simulink model "Model3"  (R2020a)
settings: Solver=VariableStepAuto  StartTime=0.0  StopTime=80  RelTol=1e-3
undefined symbols (not defined in the file): a, a0, a1, a10, a11, a12, a13, a14, a15, a16, a17, a2, a3, a4, a5, a6, a7, a8, a9, alpha, Area, b, b1, b11, b12, b2, bankingAngle, C_fuel, camber, curveCenters, Cx, Cz, distanceThreshold, g, init_vel, init_y_pos, IT, K_wear, l_f, l_r, m_fuel, mT, overlapThreshold, rho_0, rho_1, TyreContactArea, w1, w2
libraries: simulink x7
(part 1 of 2)
settings Model: PacingRate=2  Creator=carmelo  LastModifiedBy=cvalo

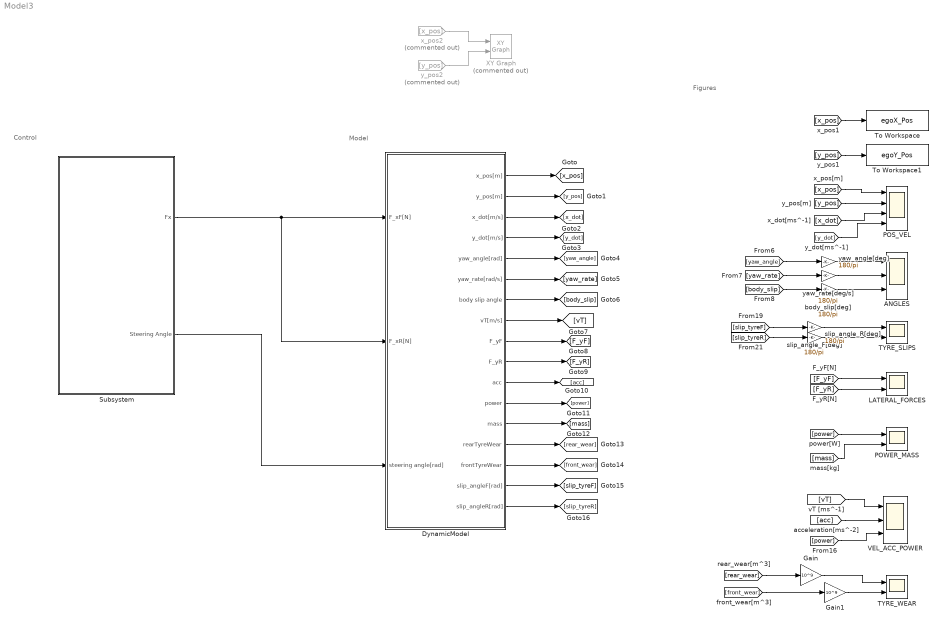
== system Model3 ==
  note: Control
  note: Model
  note: Figures
  ANGLES : Scope  NumInputPorts=3
  DynamicModel : Subsystem
  Gain : Gain  Gain=10^9
  Gain1 : Gain  Gain=10^9
  LATERAL_FORCES : Scope  NumInputPorts=2
  POS_VEL : Scope  NumInputPorts=4
  POWER_MASS : Scope  NumInputPorts=2
  Subsystem : Subsystem
  TYRE_SLIPS : Scope  NumInputPorts=2
  TYRE_WEAR : Scope  NumInputPorts=2
  To Workspace : ToWorkspace  VariableName=egoX_Pos  SampleTime=-1
      settings: Decimation=3
  To Workspace1 : ToWorkspace  VariableName=egoY_Pos  SampleTime=-1
      settings: Decimation=3
  VEL_ACC_POWER : Scope  NumInputPorts=3
  XY Graph : simulink/Sinks/XY Graph  Commented=on  xmin=-1000  xmax=1000  ymin=-1000  ymax=1000  st=-1
  body_slip[deg] : Gain  Gain=180/pi
  slip_angle_F[deg] : Gain  Gain=180/pi
  slip_angle_R[deg] : Gain  Gain=180/pi
  x_pos2 : From  Commented=on  GotoTag=x_pos
  y_pos2 : From  Commented=on  GotoTag=y_pos
  yaw_angle[deg] : Gain  Gain=180/pi
  yaw_rate[deg/s] : Gain  Gain=180/pi
  wires:
  DynamicModel/3(x_dot[m/s]) -> [x_dot]
  DynamicModel/4(y_dot[m/s]) -> [y_dot]
  DynamicModel/1(x_pos[m]) -> [x_pos]
  DynamicModel/2(y_pos[m]) -> [y_pos]
  Subsystem/1(Fx) -> DynamicModel/1(F_xF[N]), DynamicModel/2(F_xR[N])
  Subsystem/2(Steering Angle) -> DynamicModel/3(steering angle[rad])
  DynamicModel/5(yaw_angle[rad]) -> [yaw_angle]
  DynamicModel/6(yaw_rate[rad/s]) -> [yaw_rate]
  DynamicModel/7(body slip angle) -> [body_slip]
  DynamicModel/8(vT[m/s]) -> [vT]
  DynamicModel/9(F_yF) -> [F_yF]
  DynamicModel/10(F_yR) -> [F_yR]
  DynamicModel/11(acc) -> [acc]
  DynamicModel/12(power) -> [power]
  DynamicModel/13(mass) -> [mass]
  DynamicModel/15(frontTyreWear) -> [front_wear]
  DynamicModel/14(rearTyreWear) -> [rear_wear]
  DynamicModel/16(slip_angleF[rad]) -> [slip_tyreF]
  DynamicModel/17(slip_angleR[rad]) -> [slip_tyreR]
  slip_angle_R[deg]/1 -> TYRE_SLIPS/2
  [x_pos] -> POS_VEL/1
  [front_wear] -> Gain1/1
  [mass] -> POWER_MASS/2
  yaw_rate[deg/s]/1 -> ANGLES/2
  body_slip[deg]/1 -> ANGLES/3
  [yaw_angle] -> yaw_angle[deg]/1
  [y_dot] -> POS_VEL/4
  [y_pos] -> POS_VEL/2
  [yaw_rate] -> yaw_rate[deg/s]/1
  [body_slip] -> body_slip[deg]/1
  [power] -> POWER_MASS/1
  [acc] -> VEL_ACC_POWER/2
  [rear_wear] -> Gain/1
  yaw_angle[deg]/1 -> ANGLES/1
  [x_pos] -> To Workspace/1
  [F_yR] -> LATERAL_FORCES/2
  [slip_tyreR] -> slip_angle_R[deg]/1
  [y_pos] -> To Workspace1/1
  [slip_tyreF] -> slip_angle_F[deg]/1
  [F_yF] -> LATERAL_FORCES/1
  [power] -> VEL_ACC_POWER/3
  [x_dot] -> POS_VEL/3
  slip_angle_F[deg]/1 -> TYRE_SLIPS/1
  [vT] -> VEL_ACC_POWER/1
  Gain/1 -> TYRE_WEAR/1
  Gain1/1 -> TYRE_WEAR/2
  x_pos2/1 -> XY Graph/1
  y_pos2/1 -> XY Graph/2

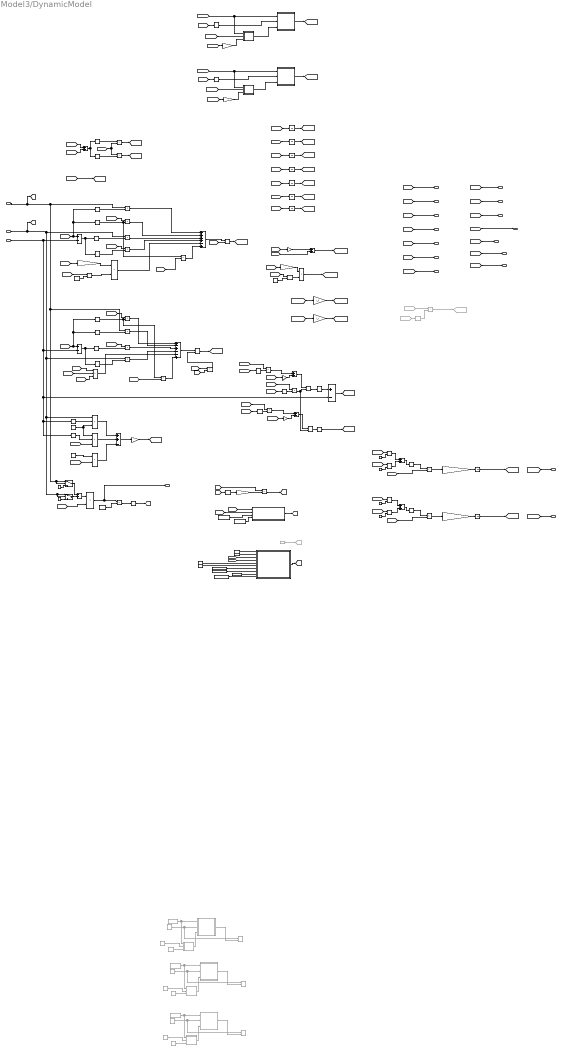
== system Model3/DynamicModel ==
  note: Wind effect
  note: DEBUG
  note: FN
  note: Fx_F
  note: Tyre wears
  note: Outputs
  note: Longitudinal velocity
  note: Outputs
  note: Tires slip angles
  note: Tire lateral forces
  note: x6_dot equation
  note: Continuos integration
  note: x4_dot equation
  note: x3_dot equation
  note: x1_dot and x2_dot equations
  note: x5_dot equation
  note: mdot
  note: vertical force
  note: Fx_R
  F_xF[N] : Inport  Unit=N
  F_xR[N] : Inport  Port=2  Unit=N
  steering angle[rad] : Inport  Port=3  Unit=rad
  Add : Sum
  Add1 : Sum
  Add2 : Sum
  Atan : Trigonometry  Operator=atan
  Atan1 : Trigonometry  Operator=atan
  Calculate Peak : Subsystem
  Calculate Peak1 : Subsystem
  Calculate Peak2 : Subsystem  Commented=on
  Calculate Peak3 : Subsystem  Commented=on
  Calculate Peak4 : Subsystem  Commented=on
  Constant : Constant  Commented=on  Value=0
  Constant1 : Constant  Value=a
  Constant10 : Constant  Value=C_fuel
  Constant{5..6,9,11..12,14} (6 alike) : Constant  Value=2
  Constant13 : Constant  Value=-5.625
  Constant15 : Constant  Commented=on  Value=7500
  Constant16 : Constant  Commented=on  Value=7500
  Constant17 : Constant  Commented=on  Value=1500
  Constant18 : Constant  Commented=on  Value=8000
  Constant19 : Constant  Value=rho_0
  Constant2 : Constant  Value=b
  Constant20 : Constant  Value=rho_1
  Constant21 : Constant  Value=distanceThreshold
  Constant22 : Constant  Value=overlapThreshold
  Constant23 : Constant  Value=curveCenters
  Constant24 : Constant  Value=alpha
  Constant25 : Constant  Commented=on  Value=rho_0
  Constant3 : Constant  Commented=on  Value=4000
  Constant32 : Constant  Value=bankingAngle
  Constant33 : Constant  Value=curveCenters
  Constant34 : Constant  Value=0
  Constant35 : Constant  Value=0
  Constant38 : Constant  Commented=on  Value=7500
  Constant4 : Constant  Commented=on  Value=1500
  Constant7 : Constant  Commented=on  Value=0
  Constant8 : Constant  Value=10
  Cos{,1..6} (7 alike) : Trigonometry  Operator=cos
  Cos7 : Trigonometry  Commented=on  Operator=cos
  Divide{,1..3} (4 alike) : Product  Inputs=*/
  FindBankingData : MATLAB Function  TreatAsAtomicUnit=on
  From37 : From  Commented=on  GotoTag=x4_vT
  From38 : From  Commented=on  GotoTag=x5_slip_angle
  Gain : Gain  Gain=g
  Gain1 : Gain  Gain=K_wear/TyreContactArea
  Gain10 : Gain  Gain=10^9
  Gain11 : Gain  Gain=10^9
  Gain2 : Gain  Gain=1/IT
  Gain21 : Gain  Gain=l_r
  Gain3 : Gain  Gain=K_wear/TyreContactArea
  Gain4 : Gain  Gain=a
  Gain5 : Gain  Gain=b
  Gain6 : Gain  Gain=Area*Cx*0.5
  Gain7 : Gain  Gain=l_f
  Gain8 : Gain  Gain=g
  Gain9 : Gain  Gain=Area*Cz*0.5
  Goto16 : Goto  Commented=on  GotoTag=longitudinal_vel
  Goto22 : Goto  Commented=on  GotoTag=rho
  Integrator{,2,4..5,7..8} (6 alike) : Integrator
  Integrator1 : Integrator  InitialCondition=init_y_pos
  Integrator3 : Integrator  InitialCondition=init_vel
  Integrator6 : Integrator  InitialCondition=mT  LimitOutput=on  UpperSaturationLimit=mT  LowerSaturationLimit=mT - m_fuel
  Minus : Sum  Inputs=+-
  Minus1 : Sum  Inputs=+-
  Minus2 : Sum  Inputs=+-
  PacejkaF : Subsystem
  PacejkaF1 : Subsystem
  PacejkaF2 : Subsystem  Commented=on
  PacejkaF3 : Subsystem  Commented=on
  PacejkaF4 : Subsystem  Commented=on
  Plus : Sum
  Plus1 : Sum  Inputs=++++-+
  Plus2 : Sum  Inputs=+-+--+
  Plus3 : Sum  Inputs=++-
  Plus4 : Sum
  Plus5 : Sum  Inputs=+-
  Plus7 : Sum
  Power{,1..5} (6 alike) : Math  Operator=pow  SaturateOnIntegerOverflow=on
  Product{,1..9,13..16,18..23,25,31,35..36} (24 alike) : Product
  Product10 : Product  Inputs=3
  Product11 : Product  Inputs=3
  Product12 : Product  Inputs=3
  Product17 : Product  Commented=on
  Ramp1 : simulink/Sources/Ramp  Commented=on  slope=0.01  start=0  InitialOutput=0
  Ramp2 : simulink/Sources/Ramp  Commented=on  slope=0.01  start=0  InitialOutput=0
  Ramp6 : simulink/Sources/Ramp  Commented=on  slope=0.01  start=0  InitialOutput=0
  Sin{,1..7,11} (9 alike) : Trigonometry
  Sqrt : Sqrt  SaturateOnIntegerOverflow=on
  Sqrt1 : Sqrt  SaturateOnIntegerOverflow=on
  Switch : Switch
  Switch1 : Switch
  Unary Minus : UnaryMinus
  Unary Minus5 : UnaryMinus
  Unary Minus6 : UnaryMinus
  WindEffect : MATLAB Function  TreatAsAtomicUnit=on
  XY Graph1 : simulink/Sinks/XY Graph  Commented=on  xmin=0  xmax=1  ymin=0  ymax=7000  st=-1
  XY Graph2 : simulink/Sinks/XY Graph  Commented=on  xmin=0  xmax=1  ymin=0  ymax=7000  st=-1
  XY Graph3 : simulink/Sinks/XY Graph  Commented=on  xmin=0  xmax=1  ymin=0  ymax=7000  st=-1
  x_pos[m] : Outport  Unit=m
  y_pos[m] : Outport  Port=2  Unit=m
  x_dot[m/s] : Outport  Port=3  Unit=m/s
  y_dot[m/s] : Outport  Port=4  Unit=m/s
  yaw_angle[rad] : Outport  Port=5  Unit=rad
  yaw_rate[rad/s] : Outport  Port=6  Unit=rad/s
  body slip angle : Outport  Port=7  Unit=rad
  vT[m/s] : Outport  Port=8  Unit=m/s
  F_yF : Outport  Port=9  Unit=N
  F_yR : Outport  Port=10  Unit=N
  acc : Outport  Port=11  Unit=m/s^2
  power : Outport  Port=12  Unit=watt
  mass : Outport  Port=13  Unit=kg
  rearTyreWear : Outport  Port=14  Unit=m^3
  frontTyreWear : Outport  Port=15  Unit=m^3
  slip_angleF[rad] : Outport  Port=16  Unit=rad
  slip_angleR[rad] : Outport  Port=17  Unit=rad
  wires:
  [x5_slip_angle] -> Sin7/1
  [x4_vT] -> Product16/1
  Atan/1 -> Minus2/1
  Product17/1 -> Goto16/1
  [x1_x_pos] -> x_pos[m]/1
  [x6_yaw_rate] -> Gain4/1
  [F_yR] -> Product13/2
  Sin/1 -> Product1/2
  Integrator3/1 -> [x4_vT]
  Cos7/1 -> Product17/2
  Sin2/1 -> Product35/1, Product4/2
  Product4/1 -> Plus1/2
  [x3_dot] -> Integrator2/1
  Divide1/1 -> Atan1/1
  Product2/1 -> Plus1/3
  [F_yF] -> Product6/1
  Product14/1 -> Divide/2, Divide1/2
  [x5_slip_angle] -> Sin2/1, Cos2/1, Minus/1
  Minus2/1 -> [slip_angle_F]
  Cos2/1 -> Product3/2
  [x5_slip_angle] -> Plus/2
  Sin7/1 -> Product16/2
  Integrator5/1 -> [x6_yaw_rate]
  [x4_dot] -> Integrator3/1
  Product/1 -> [x1_dot]
  [x3_yaw_angle] -> yaw_angle[rad]/1
  [x1_dot] -> x_dot[m/s]/1
  Constant2/1 -> Product13/1
  Cos3/1 -> Product6/2
  [x2_dot] -> Integrator1/1
  Minus/1 -> Sin1/1, Cos1/1
  [x6_dot] -> Integrator5/1
  Integrator2/1 -> [x3_yaw_angle]
  Gain4/1 -> Plus4/2
  [x2_y_pos] -> y_pos[m]/1
  Cos1/1 -> Product2/2
  Gain2/1 -> [x6_dot]
  [x4_vT] -> Product10/2
  [x6_yaw_rate] -> [x3_dot]
  [F_yF] -> Product5/1
  [x3_yaw_angle] -> Plus/1
  [x6_yaw_rate] -> yaw_rate[rad/s]/1
  [F_yR] -> Product4/1
  [x4_vT] -> Product15/1
  [x4_vT] -> vT[m/s]/1
  [x5_slip_angle] -> Sin6/1
  Product11/1 -> Plus3/1
  [F_yR] -> Product7/1
  Atan1/1 -> [slip_angle_R]
  Divide/1 -> Atan/1
  [x4_vT] -> Product1/1, Product/2
  Product1/1 -> [x2_dot]
  Cos4/1 -> Product36/1, Product7/2
  Sin5/1 -> Product11/2
  Plus5/1 -> Divide1/1
  [x5_slip_angle] -> Cos6/1
  Sin4/1 -> Product8/2
  [x6_yaw_rate] -> Product10/3
  Cos5/1 -> Product12/2
  Plus3/1 -> Gain2/1
  Cos/1 -> Product/1
  Product13/1 -> Plus3/3
  Cos6/1 -> Product14/2
  Integrator/1 -> [x1_x_pos]
  Plus/1 -> Cos/1, Sin/1
  Product12/1 -> Plus3/2
  Product5/1 -> Plus1/4
  steering angle[rad]/1 -> Minus2/2, Cos5/1, Sin5/1, Minus1/2, Minus/2
  Product15/1 -> Plus4/1
  [x5_dot] -> Integrator4/1
  Product9/1 -> Plus2/4
  Product16/1 -> Plus5/1
  [x4_vT] -> Product14/1
  [mT] -> Product10/1
  From37/1 -> Product17/1
  Sin3/1 -> Product9/2
  Plus2/1 -> Divide2/1
  Product6/1 -> Plus2/3
  [x5_slip_angle] -> Sin4/1, Cos4/1, Minus1/1
  Constant1/1 -> Product11/3, Product12/1
  Divide2/1 -> [x5_dot]
  Integrator1/1 -> [x2_y_pos]
  [F_yF] -> Product12/3
  Minus1/1 -> Sin3/1, Cos3/1
  Product10/1 -> Plus2/5
  Product7/1 -> Plus2/1
  From38/1 -> Cos7/1
  Sin1/1 -> Product5/2
  [x6_yaw_rate] -> Gain5/1
  [x1_dot] -> Integrator/1
  [x2_dot] -> y_dot[m/s]/1
  Product3/1 -> Plus1/1
  Sin6/1 -> Product15/2
  Integrator4/1 -> [x5_slip_angle]
  Product8/1 -> Plus2/2
  Plus4/1 -> Divide/1
  Gain5/1 -> Plus5/2
  Divide3/1 -> [x4_dot]
  Plus1/1 -> Divide3/1
  [F_yF] -> F_yF/1
  [F_yR] -> F_yR/1
  [x5_slip_angle] -> body slip angle/1
  [x4_dot] -> acc/1
  Product18/1 -> Divide2/2
  [mT] -> Product18/1
  [x4_vT] -> Product18/2
  [x4_vT] -> Power/1
  Product19/1 -> Plus1/5
  [rho] -> Gain6/1
  Constant6/1 -> Power/2
  Gain6/1 -> Product19/1
  Power/1 -> Product19/2
  Product21/1 -> Product22/1, power/1
  Add/1 -> Product21/1
  Constant10/1 -> Product22/2
  F_xF[N]/1 -> Product9/1, Switch1/1, Switch1/2, Product11/1, Product2/1, [F_xF]
  [x4_vT] -> Product21/2
  Plus7/1 -> [F_z]
  [F_lift] -> Plus7/2
  [mT] -> Gain8/1
  Product22/1 -> Unary Minus/1
  Unary Minus/1 -> [mTdot]
  [mTdot] -> Integrator6/1
  Integrator6/1 -> [mT]
  [mT] -> mass/1
  [mT] -> Divide3/2
  [F_zR] -> Product31/2
  Product31/1 -> Gain1/1
  Gain1/1 -> Integrator7/1
  Integrator7/1 -> [RearWear]
  [RearWear] -> rearTyreWear/1
  [FrontWear] -> frontTyreWear/1
  Integrator8/1 -> [FrontWear]
  [FNX] -> Product35/2
  Product35/1 -> Plus1/6
  [FNX] -> Product36/2
  Product36/1 -> Plus2/6
  Sin11/1 -> Gain/1
  [gamma] -> Sin11/1
  Power2/1 -> Product23/2
  Gain9/1 -> Product23/1
  Constant12/1 -> Power2/2
  [x4_vT] -> Power2/1
  [rho] -> Gain9/1
  Product23/1 -> [F_lift]
  FindBankingData/1(res) -> [gamma]
  [x1_x_pos] -> FindBankingData/1(x)
  [x2_y_pos] -> FindBankingData/2(y)
  Constant33/1 -> FindBankingData/3(curveCenters)
  Constant32/1 -> FindBankingData/4(bankingAngle)
  [F_z] -> Gain7/1
  Gain7/1 -> [F_zF]
  [F_z] -> Gain21/1
  Gain21/1 -> [F_zR]
  Gain/1 -> Product25/2
  F_xR[N]/1 -> Product3/1, Switch/2, Switch/1, Product8/1, [F_xR]
  Constant34/1 -> Switch/3
  Switch/1 -> Add/1
  Switch1/1 -> Add/2
  Constant35/1 -> Switch1/3
  Sqrt/1 -> Product31/1
  Add1/1 -> Sqrt/1
  [F_xR] -> Power1/1
  Constant5/1 -> Power1/2
  [F_yR] -> Power4/1
  Constant9/1 -> Power4/2
  Power4/1 -> Add1/2
  Power1/1 -> Add1/1
  [F_zF] -> Product20/2
  [F_xF] -> Power3/1
  Product20/1 -> Gain3/1
  Add2/1 -> Sqrt1/1
  [F_yF] -> Power5/1
  Power3/1 -> Add2/1
  Power5/1 -> Add2/2
  Constant11/1 -> Power3/2
  Gain3/1 -> Integrator8/1
  Constant14/1 -> Power5/2
  Sqrt1/1 -> Product20/1
  Gain8/1 -> Plus7/1
  [mT] -> Product25/1
  Product25/1 -> [FNX]
  Constant38/1 -> Calculate Peak2/1(Fz), PacejkaF2/1(Fz[N])
  Ramp6/1 -> XY Graph1/1, PacejkaF2/2(slip)
  PacejkaF1/1(Fy) -> [F_yR]
  PacejkaF/1(Fy) -> [F_yF]
  [slip_angle_R] -> Unary Minus5/1
  Unary Minus5/1 -> PacejkaF1/2(slip)
  [slip_angle_F] -> Unary Minus6/1
  Unary Minus6/1 -> PacejkaF/2(slip)
  [F_zF] -> Calculate Peak/1(Fz), PacejkaF/1(Fz[N])
  Calculate Peak/1(Peak) -> PacejkaF/3(D)
  [F_xF] -> Calculate Peak/2(Fx)
  [FrontWear] -> Gain10/1
  Gain10/1 -> Calculate Peak/3(Wear)
  [RearWear] -> Gain11/1
  [F_xR] -> Calculate Peak1/2(Fx)
  [F_zR] -> Calculate Peak1/1(Fz), PacejkaF1/1(Fz[N])
  Calculate Peak1/1(Peak) -> PacejkaF1/3(D)
  Gain11/1 -> Calculate Peak1/3(Wear)
  PacejkaF2/1(Fy) -> XY Graph1/2
  Constant/1 -> Calculate Peak2/3(Wear)
  Constant3/1 -> Calculate Peak2/2(Fx)
  Calculate Peak2/1(Peak) -> PacejkaF2/3(D)
  Constant15/1 -> Calculate Peak3/1(Fz), PacejkaF3/1(Fz[N])
  Constant4/1 -> Calculate Peak3/2(Fx)
  Calculate Peak3/1(Peak) -> PacejkaF3/3(D)
  PacejkaF3/1(Fy) -> XY Graph2/2
  Constant7/1 -> Calculate Peak3/3(Wear)
  Ramp1/1 -> XY Graph2/1, PacejkaF3/2(slip)
  Constant17/1 -> Calculate Peak4/2(Fx)
  Ramp2/1 -> XY Graph3/1, PacejkaF4/2(slip)
  PacejkaF4/1(Fy) -> XY Graph3/2
  Constant16/1 -> Calculate Peak4/1(Fz), PacejkaF4/1(Fz[N])
  Calculate Peak4/1(Peak) -> PacejkaF4/3(D)
  Constant18/1 -> Calculate Peak4/3(Wear)
  WindEffect/1(aerodynamic_coeff) -> [rho]
  Constant19/1 -> WindEffect/1(rho_0)
  Constant20/1 -> WindEffect/2(rho_1)
  [x2_y_pos] -> WindEffect/4(ego_y)
  [x1_x_pos] -> WindEffect/3(ego_x)
  [slip_angle_F] -> slip_angleF[rad]/1
  [slip_angle_R] -> slip_angleR[rad]/1
  Constant8/1 -> WindEffect/5(opp_x)
  Constant13/1 -> WindEffect/6(opp_y)
  Constant21/1 -> WindEffect/7(distanceThreshold)
  Constant22/1 -> WindEffect/8(overlapThreshold)
  Constant24/1 -> WindEffect/9(alpha)
  Constant23/1 -> WindEffect/10(curveCenters)
  Constant25/1 -> Goto22/1

== system Model3/Subsystem ==
  Digital Clock : DigitalClock
  MATLAB Function : MATLAB Function  TreatAsAtomicUnit=on
  MATLAB Function1 : MATLAB Function  TreatAsAtomicUnit=on
  Fx : Outport  Unit=N
  Steering Angle : Outport  Port=2  Unit=rad
  wires:
  Digital Clock/1 -> MATLAB Function/1(clock), MATLAB Function1/1(clock)
  MATLAB Function/1(force) -> Fx/1
  MATLAB Function1/1(steer) -> Steering Angle/1

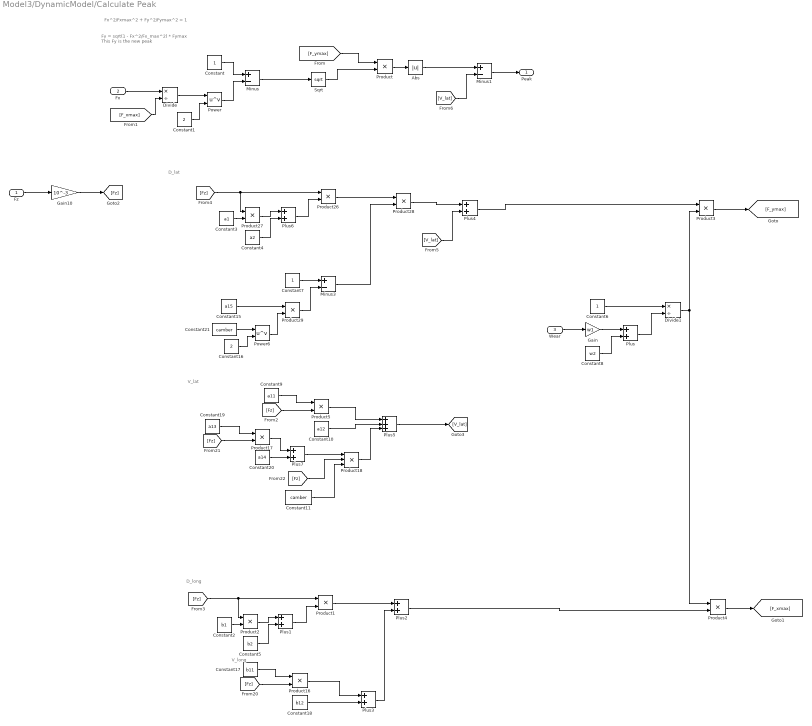
== system Model3/DynamicModel/Calculate Peak ==
  note: V_lat
  note: D_lat
  note: D_long
  note: V_long
  note: Fy = sqrt(1 - Fx^2/Fx_max^2) * Fymax
      |
      | This Fy is the new peak
  note: Fx^2/Fxmax^2 + Fy^2/Fymax^2 = 1
  Fz : Inport  Unit=N
  Fx : Inport  Port=2  Unit=N
  Wear : Inport  Port=3
  Abs : Abs
  Constant : Constant
  Constant1 : Constant  Value=2
  Constant10 : Constant  Value=a12
  Constant11 : Constant  Value=camber
  Constant15 : Constant  Value=a15
  Constant16 : Constant  Value=2
  Constant17 : Constant  Value=b11
  Constant18 : Constant  Value=b12
  Constant19 : Constant  Value=a13
  Constant2 : Constant  Value=b1
  Constant20 : Constant  Value=a14
  Constant21 : Constant  Value=camber
  Constant3 : Constant  Value=a1
  Constant4 : Constant  Value=a2
  Constant5 : Constant  Value=b2
  Constant6 : Constant
  Constant7 : Constant
  Constant8 : Constant  Value=w2
  Constant9 : Constant  Value=a11
  Divide : Product  Inputs=*/
  Divide1 : Product  Inputs=*/
  Gain : Gain  Gain=w1
  Gain10 : Gain  Gain=10^-3
  Minus : Sum  Inputs=+-
  Minus1 : Sum  Inputs=+-
  Minus3 : Sum  Inputs=+-
  Plus{,1..4,6..7} (7 alike) : Sum
  Plus5 : Sum  Inputs=+++
  Power : Math  Operator=pow  SaturateOnIntegerOverflow=on
  Power6 : Math  Operator=pow  SaturateOnIntegerOverflow=on
  Product{,1..5,16..17,26..29} (12 alike) : Product
  Product18 : Product  Inputs=3
  Sqrt : Sqrt  SaturateOnIntegerOverflow=on
  Peak : Outport
  wires:
  Minus3/1 -> Product28/2
  Constant7/1 -> Minus3/1
  Constant16/1 -> Power6/2
  Product27/1 -> Plus6/1
  Constant21/1 -> Power6/1
  Product29/1 -> Minus3/2
  Product26/1 -> Product28/1
  Constant15/1 -> Product29/1
  Power6/1 -> Product29/2
  Plus6/1 -> Product26/2
  [Fz] -> Product27/1, Product26/1
  Constant3/1 -> Product27/2
  Constant4/1 -> Plus6/2
  Product/1 -> Abs/1
  [F_ymax] -> Product/1
  Sqrt/1 -> Product/2
  Constant/1 -> Minus/1
  Minus/1 -> Sqrt/1
  Fx/1 -> Divide/1
  Divide/1 -> Power/1
  Power/1 -> Minus/2
  Constant1/1 -> Power/2
  [F_xmax] -> Divide/2
  Product1/1 -> Plus2/1
  [Fz] -> Product2/1, Product1/1
  Plus1/1 -> Product1/2
  Product2/1 -> Plus1/1
  Constant5/1 -> Plus1/2
  Constant2/1 -> Product2/2
  Constant17/1 -> Product16/1
  Product16/1 -> Plus3/1
  [Fz] -> Product16/2
  Constant18/1 -> Plus3/2
  Plus3/1 -> Plus2/2
  Constant6/1 -> Divide1/1
  Plus/1 -> Divide1/2
  Constant8/1 -> Plus/2
  Gain/1 -> Plus/1
  Wear/1 -> Gain/1
  Divide1/1 -> Product4/1, Product3/2
  Product3/1 -> [F_ymax]
  Product4/1 -> [F_xmax]
  Plus2/1 -> Product4/2
  Product28/1 -> Plus4/1
  Plus4/1 -> Product3/1
  Constant10/1 -> Plus5/2
  Plus7/1 -> Product18/1
  [Fz] -> Product17/2
  Constant20/1 -> Plus7/2
  Product18/1 -> Plus5/3
  Constant19/1 -> Product17/1
  Product17/1 -> Plus7/1
  Constant11/1 -> Product18/3
  Constant9/1 -> Product5/1
  Product5/1 -> Plus5/1
  [Fz] -> Product5/2
  [Fz] -> Product18/2
  Fz/1 -> Gain10/1
  Gain10/1 -> [Fz]
  Plus5/1 -> [V_lat]
  [V_lat] -> Plus4/2
  Abs/1 -> Minus1/1
  Minus1/1 -> Peak/1
  [V_lat] -> Minus1/2

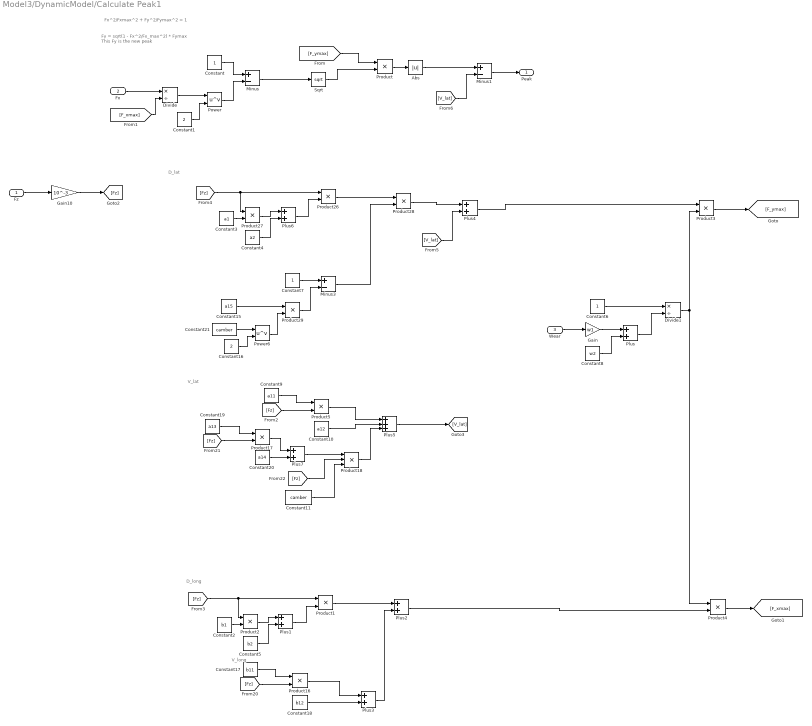
== system Model3/DynamicModel/Calculate Peak1 ==
  note: V_lat
  note: D_lat
  note: D_long
  note: V_long
  note: Fy = sqrt(1 - Fx^2/Fx_max^2) * Fymax
      |
      | This Fy is the new peak
  note: Fx^2/Fxmax^2 + Fy^2/Fymax^2 = 1
  Fz : Inport  Unit=N
  Fx : Inport  Port=2  Unit=N
  Wear : Inport  Port=3
  Abs : Abs
  Constant : Constant
  Constant1 : Constant  Value=2
  Constant10 : Constant  Value=a12
  Constant11 : Constant  Value=camber
  Constant15 : Constant  Value=a15
  Constant16 : Constant  Value=2
  Constant17 : Constant  Value=b11
  Constant18 : Constant  Value=b12
  Constant19 : Constant  Value=a13
  Constant2 : Constant  Value=b1
  Constant20 : Constant  Value=a14
  Constant21 : Constant  Value=camber
  Constant3 : Constant  Value=a1
  Constant4 : Constant  Value=a2
  Constant5 : Constant  Value=b2
  Constant6 : Constant
  Constant7 : Constant
  Constant8 : Constant  Value=w2
  Constant9 : Constant  Value=a11
  Divide : Product  Inputs=*/
  Divide1 : Product  Inputs=*/
  Gain : Gain  Gain=w1
  Gain10 : Gain  Gain=10^-3
  Minus : Sum  Inputs=+-
  Minus1 : Sum  Inputs=+-
  Minus3 : Sum  Inputs=+-
  Plus{,1..4,6..7} (7 alike) : Sum
  Plus5 : Sum  Inputs=+++
  Power : Math  Operator=pow  SaturateOnIntegerOverflow=on
  Power6 : Math  Operator=pow  SaturateOnIntegerOverflow=on
  Product{,1..5,16..17,26..29} (12 alike) : Product
  Product18 : Product  Inputs=3
  Sqrt : Sqrt  SaturateOnIntegerOverflow=on
  Peak : Outport
  wires:
  Minus3/1 -> Product28/2
  Constant7/1 -> Minus3/1
  Constant16/1 -> Power6/2
  Product27/1 -> Plus6/1
  Constant21/1 -> Power6/1
  Product29/1 -> Minus3/2
  Product26/1 -> Product28/1
  Constant15/1 -> Product29/1
  Power6/1 -> Product29/2
  Plus6/1 -> Product26/2
  [Fz] -> Product27/1, Product26/1
  Constant3/1 -> Product27/2
  Constant4/1 -> Plus6/2
  Product/1 -> Abs/1
  [F_ymax] -> Product/1
  Sqrt/1 -> Product/2
  Constant/1 -> Minus/1
  Minus/1 -> Sqrt/1
  Fx/1 -> Divide/1
  Divide/1 -> Power/1
  Power/1 -> Minus/2
  Constant1/1 -> Power/2
  [F_xmax] -> Divide/2
  Product1/1 -> Plus2/1
  [Fz] -> Product2/1, Product1/1
  Plus1/1 -> Product1/2
  Product2/1 -> Plus1/1
  Constant5/1 -> Plus1/2
  Constant2/1 -> Product2/2
  Constant17/1 -> Product16/1
  Product16/1 -> Plus3/1
  [Fz] -> Product16/2
  Constant18/1 -> Plus3/2
  Plus3/1 -> Plus2/2
  Constant6/1 -> Divide1/1
  Plus/1 -> Divide1/2
  Constant8/1 -> Plus/2
  Gain/1 -> Plus/1
  Wear/1 -> Gain/1
  Divide1/1 -> Product4/1, Product3/2
  Product3/1 -> [F_ymax]
  Product4/1 -> [F_xmax]
  Plus2/1 -> Product4/2
  Product28/1 -> Plus4/1
  Plus4/1 -> Product3/1
  Constant10/1 -> Plus5/2
  Plus7/1 -> Product18/1
  [Fz] -> Product17/2
  Constant20/1 -> Plus7/2
  Product18/1 -> Plus5/3
  Constant19/1 -> Product17/1
  Product17/1 -> Plus7/1
  Constant11/1 -> Product18/3
  Constant9/1 -> Product5/1
  Product5/1 -> Plus5/1
  [Fz] -> Product5/2
  [Fz] -> Product18/2
  Fz/1 -> Gain10/1
  Gain10/1 -> [Fz]
  Plus5/1 -> [V_lat]
  [V_lat] -> Plus4/2
  Abs/1 -> Minus1/1
  Minus1/1 -> Peak/1
  [V_lat] -> Minus1/2

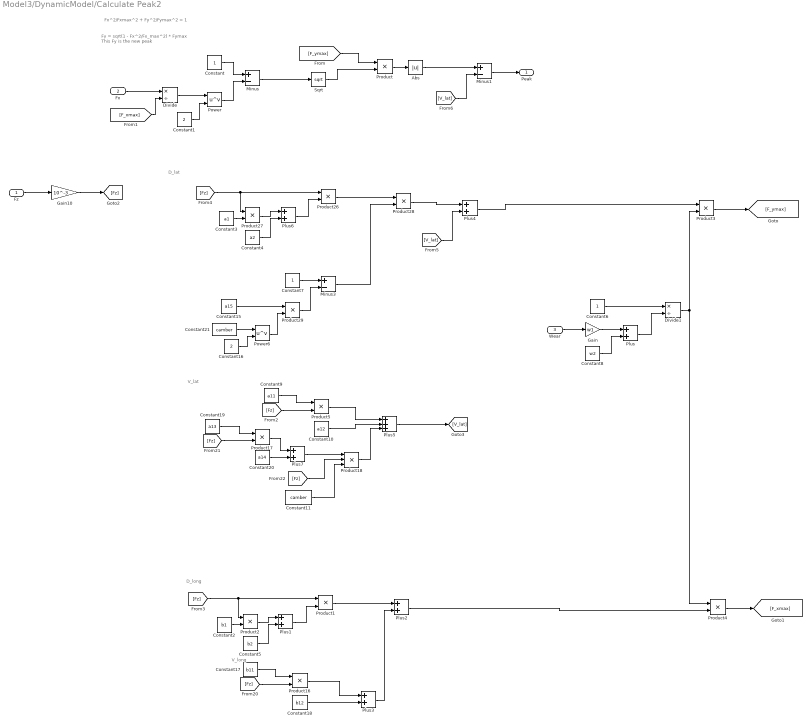
== system Model3/DynamicModel/Calculate Peak2 ==
  note: V_lat
  note: D_lat
  note: D_long
  note: V_long
  note: Fy = sqrt(1 - Fx^2/Fx_max^2) * Fymax
      |
      | This Fy is the new peak
  note: Fx^2/Fxmax^2 + Fy^2/Fymax^2 = 1
  Fz : Inport  Unit=N
  Fx : Inport  Port=2  Unit=N
  Wear : Inport  Port=3
  Abs : Abs
  Constant : Constant
  Constant1 : Constant  Value=2
  Constant10 : Constant  Value=a12
  Constant11 : Constant  Value=camber
  Constant15 : Constant  Value=a15
  Constant16 : Constant  Value=2
  Constant17 : Constant  Value=b11
  Constant18 : Constant  Value=b12
  Constant19 : Constant  Value=a13
  Constant2 : Constant  Value=b1
  Constant20 : Constant  Value=a14
  Constant21 : Constant  Value=camber
  Constant3 : Constant  Value=a1
  Constant4 : Constant  Value=a2
  Constant5 : Constant  Value=b2
  Constant6 : Constant
  Constant7 : Constant
  Constant8 : Constant  Value=w2
  Constant9 : Constant  Value=a11
  Divide : Product  Inputs=*/
  Divide1 : Product  Inputs=*/
  Gain : Gain  Gain=w1
  Gain10 : Gain  Gain=10^-3
  Minus : Sum  Inputs=+-
  Minus1 : Sum  Inputs=+-
  Minus3 : Sum  Inputs=+-
  Plus{,1..4,6..7} (7 alike) : Sum
  Plus5 : Sum  Inputs=+++
  Power : Math  Operator=pow  SaturateOnIntegerOverflow=on
  Power6 : Math  Operator=pow  SaturateOnIntegerOverflow=on
  Product{,1..5,16..17,26..29} (12 alike) : Product
  Product18 : Product  Inputs=3
  Sqrt : Sqrt  SaturateOnIntegerOverflow=on
  Peak : Outport
  wires:
  Minus3/1 -> Product28/2
  Constant7/1 -> Minus3/1
  Constant16/1 -> Power6/2
  Product27/1 -> Plus6/1
  Constant21/1 -> Power6/1
  Product29/1 -> Minus3/2
  Product26/1 -> Product28/1
  Constant15/1 -> Product29/1
  Power6/1 -> Product29/2
  Plus6/1 -> Product26/2
  [Fz] -> Product27/1, Product26/1
  Constant3/1 -> Product27/2
  Constant4/1 -> Plus6/2
  Product/1 -> Abs/1
  [F_ymax] -> Product/1
  Sqrt/1 -> Product/2
  Constant/1 -> Minus/1
  Minus/1 -> Sqrt/1
  Fx/1 -> Divide/1
  Divide/1 -> Power/1
  Power/1 -> Minus/2
  Constant1/1 -> Power/2
  [F_xmax] -> Divide/2
  Product1/1 -> Plus2/1
  [Fz] -> Product2/1, Product1/1
  Plus1/1 -> Product1/2
  Product2/1 -> Plus1/1
  Constant5/1 -> Plus1/2
  Constant2/1 -> Product2/2
  Constant17/1 -> Product16/1
  Product16/1 -> Plus3/1
  [Fz] -> Product16/2
  Constant18/1 -> Plus3/2
  Plus3/1 -> Plus2/2
  Constant6/1 -> Divide1/1
  Plus/1 -> Divide1/2
  Constant8/1 -> Plus/2
  Gain/1 -> Plus/1
  Wear/1 -> Gain/1
  Divide1/1 -> Product4/1, Product3/2
  Product3/1 -> [F_ymax]
  Product4/1 -> [F_xmax]
  Plus2/1 -> Product4/2
  Product28/1 -> Plus4/1
  Plus4/1 -> Product3/1
  Constant10/1 -> Plus5/2
  Plus7/1 -> Product18/1
  [Fz] -> Product17/2
  Constant20/1 -> Plus7/2
  Product18/1 -> Plus5/3
  Constant19/1 -> Product17/1
  Product17/1 -> Plus7/1
  Constant11/1 -> Product18/3
  Constant9/1 -> Product5/1
  Product5/1 -> Plus5/1
  [Fz] -> Product5/2
  [Fz] -> Product18/2
  Fz/1 -> Gain10/1
  Gain10/1 -> [Fz]
  Plus5/1 -> [V_lat]
  [V_lat] -> Plus4/2
  Abs/1 -> Minus1/1
  Minus1/1 -> Peak/1
  [V_lat] -> Minus1/2

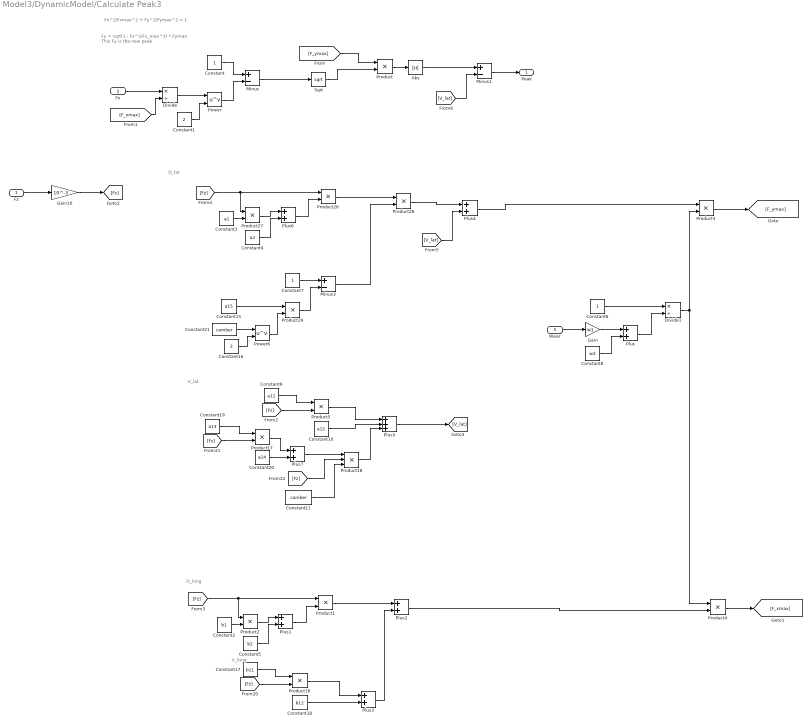
== system Model3/DynamicModel/Calculate Peak3 ==
  note: V_lat
  note: D_lat
  note: D_long
  note: V_long
  note: Fy = sqrt(1 - Fx^2/Fx_max^2) * Fymax
      |
      | This Fy is the new peak
  note: Fx^2/Fxmax^2 + Fy^2/Fymax^2 = 1
  Fz : Inport  Unit=N
  Fx : Inport  Port=2  Unit=N
  Wear : Inport  Port=3
  Abs : Abs
  Constant : Constant
  Constant1 : Constant  Value=2
  Constant10 : Constant  Value=a12
  Constant11 : Constant  Value=camber
  Constant15 : Constant  Value=a15
  Constant16 : Constant  Value=2
  Constant17 : Constant  Value=b11
  Constant18 : Constant  Value=b12
  Constant19 : Constant  Value=a13
  Constant2 : Constant  Value=b1
  Constant20 : Constant  Value=a14
  Constant21 : Constant  Value=camber
  Constant3 : Constant  Value=a1
  Constant4 : Constant  Value=a2
  Constant5 : Constant  Value=b2
  Constant6 : Constant
  Constant7 : Constant
  Constant8 : Constant  Value=w2
  Constant9 : Constant  Value=a11
  Divide : Product  Inputs=*/
  Divide1 : Product  Inputs=*/
  Gain : Gain  Gain=w1
  Gain10 : Gain  Gain=10^-3
  Minus : Sum  Inputs=+-
  Minus1 : Sum  Inputs=+-
  Minus3 : Sum  Inputs=+-
  Plus{,1..4,6..7} (7 alike) : Sum
  Plus5 : Sum  Inputs=+++
  Power : Math  Operator=pow  SaturateOnIntegerOverflow=on
  Power6 : Math  Operator=pow  SaturateOnIntegerOverflow=on
  Product{,1..5,16..17,26..29} (12 alike) : Product
  Product18 : Product  Inputs=3
  Sqrt : Sqrt  SaturateOnIntegerOverflow=on
  Peak : Outport
  wires:
  Minus3/1 -> Product28/2
  Constant7/1 -> Minus3/1
  Constant16/1 -> Power6/2
  Product27/1 -> Plus6/1
  Constant21/1 -> Power6/1
  Product29/1 -> Minus3/2
  Product26/1 -> Product28/1
  Constant15/1 -> Product29/1
  Power6/1 -> Product29/2
  Plus6/1 -> Product26/2
  [Fz] -> Product27/1, Product26/1
  Constant3/1 -> Product27/2
  Constant4/1 -> Plus6/2
  Product/1 -> Abs/1
  [F_ymax] -> Product/1
  Sqrt/1 -> Product/2
  Constant/1 -> Minus/1
  Minus/1 -> Sqrt/1
  Fx/1 -> Divide/1
  Divide/1 -> Power/1
  Power/1 -> Minus/2
  Constant1/1 -> Power/2
  [F_xmax] -> Divide/2
  Product1/1 -> Plus2/1
  [Fz] -> Product2/1, Product1/1
  Plus1/1 -> Product1/2
  Product2/1 -> Plus1/1
  Constant5/1 -> Plus1/2
  Constant2/1 -> Product2/2
  Constant17/1 -> Product16/1
  Product16/1 -> Plus3/1
  [Fz] -> Product16/2
  Constant18/1 -> Plus3/2
  Plus3/1 -> Plus2/2
  Constant6/1 -> Divide1/1
  Plus/1 -> Divide1/2
  Constant8/1 -> Plus/2
  Gain/1 -> Plus/1
  Wear/1 -> Gain/1
  Divide1/1 -> Product4/1, Product3/2
  Product3/1 -> [F_ymax]
  Product4/1 -> [F_xmax]
  Plus2/1 -> Product4/2
  Product28/1 -> Plus4/1
  Plus4/1 -> Product3/1
  Constant10/1 -> Plus5/2
  Plus7/1 -> Product18/1
  [Fz] -> Product17/2
  Constant20/1 -> Plus7/2
  Product18/1 -> Plus5/3
  Constant19/1 -> Product17/1
  Product17/1 -> Plus7/1
  Constant11/1 -> Product18/3
  Constant9/1 -> Product5/1
  Product5/1 -> Plus5/1
  [Fz] -> Product5/2
  [Fz] -> Product18/2
  Fz/1 -> Gain10/1
  Gain10/1 -> [Fz]
  Plus5/1 -> [V_lat]
  [V_lat] -> Plus4/2
  Abs/1 -> Minus1/1
  Minus1/1 -> Peak/1
  [V_lat] -> Minus1/2

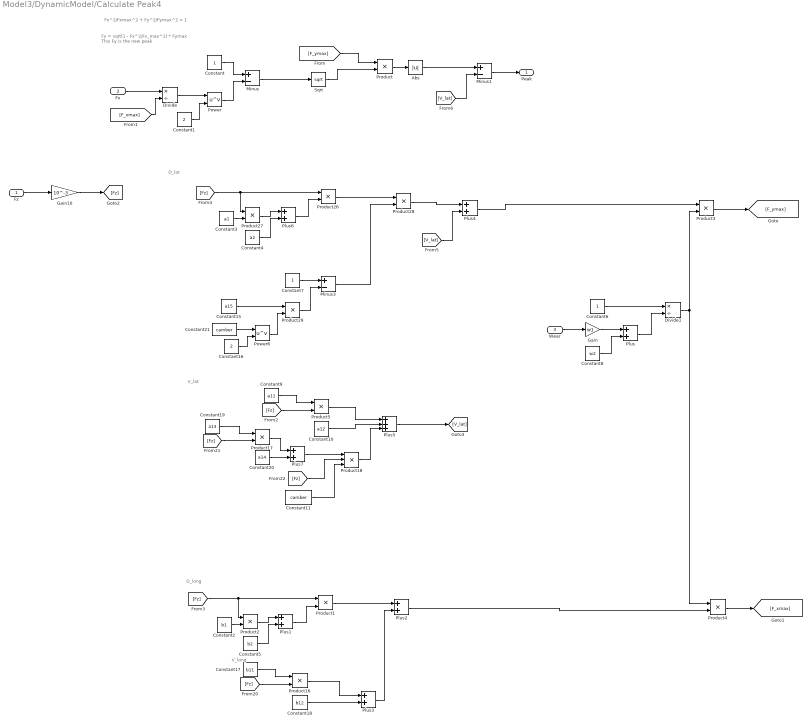
== system Model3/DynamicModel/Calculate Peak4 ==
  note: V_lat
  note: D_lat
  note: D_long
  note: V_long
  note: Fy = sqrt(1 - Fx^2/Fx_max^2) * Fymax
      |
      | This Fy is the new peak
  note: Fx^2/Fxmax^2 + Fy^2/Fymax^2 = 1
  Fz : Inport  Unit=N
  Fx : Inport  Port=2  Unit=N
  Wear : Inport  Port=3
  Abs : Abs
  Constant : Constant
  Constant1 : Constant  Value=2
  Constant10 : Constant  Value=a12
  Constant11 : Constant  Value=camber
  Constant15 : Constant  Value=a15
  Constant16 : Constant  Value=2
  Constant17 : Constant  Value=b11
  Constant18 : Constant  Value=b12
  Constant19 : Constant  Value=a13
  Constant2 : Constant  Value=b1
  Constant20 : Constant  Value=a14
  Constant21 : Constant  Value=camber
  Constant3 : Constant  Value=a1
  Constant4 : Constant  Value=a2
  Constant5 : Constant  Value=b2
  Constant6 : Constant
  Constant7 : Constant
  Constant8 : Constant  Value=w2
  Constant9 : Constant  Value=a11
  Divide : Product  Inputs=*/
  Divide1 : Product  Inputs=*/
  Gain : Gain  Gain=w1
  Gain10 : Gain  Gain=10^-3
  Minus : Sum  Inputs=+-
  Minus1 : Sum  Inputs=+-
  Minus3 : Sum  Inputs=+-
  Plus{,1..4,6..7} (7 alike) : Sum
  Plus5 : Sum  Inputs=+++
  Power : Math  Operator=pow  SaturateOnIntegerOverflow=on
  Power6 : Math  Operator=pow  SaturateOnIntegerOverflow=on
  Product{,1..5,16..17,26..29} (12 alike) : Product
  Product18 : Product  Inputs=3
  Sqrt : Sqrt  SaturateOnIntegerOverflow=on
  Peak : Outport
  wires:
  Minus3/1 -> Product28/2
  Constant7/1 -> Minus3/1
  Constant16/1 -> Power6/2
  Product27/1 -> Plus6/1
  Constant21/1 -> Power6/1
  Product29/1 -> Minus3/2
  Product26/1 -> Product28/1
  Constant15/1 -> Product29/1
  Power6/1 -> Product29/2
  Plus6/1 -> Product26/2
  [Fz] -> Product27/1, Product26/1
  Constant3/1 -> Product27/2
  Constant4/1 -> Plus6/2
  Product/1 -> Abs/1
  [F_ymax] -> Product/1
  Sqrt/1 -> Product/2
  Constant/1 -> Minus/1
  Minus/1 -> Sqrt/1
  Fx/1 -> Divide/1
  Divide/1 -> Power/1
  Power/1 -> Minus/2
  Constant1/1 -> Power/2
  [F_xmax] -> Divide/2
  Product1/1 -> Plus2/1
  [Fz] -> Product2/1, Product1/1
  Plus1/1 -> Product1/2
  Product2/1 -> Plus1/1
  Constant5/1 -> Plus1/2
  Constant2/1 -> Product2/2
  Constant17/1 -> Product16/1
  Product16/1 -> Plus3/1
  [Fz] -> Product16/2
  Constant18/1 -> Plus3/2
  Plus3/1 -> Plus2/2
  Constant6/1 -> Divide1/1
  Plus/1 -> Divide1/2
  Constant8/1 -> Plus/2
  Gain/1 -> Plus/1
  Wear/1 -> Gain/1
  Divide1/1 -> Product4/1, Product3/2
  Product3/1 -> [F_ymax]
  Product4/1 -> [F_xmax]
  Plus2/1 -> Product4/2
  Product28/1 -> Plus4/1
  Plus4/1 -> Product3/1
  Constant10/1 -> Plus5/2
  Plus7/1 -> Product18/1
  [Fz] -> Product17/2
  Constant20/1 -> Plus7/2
  Product18/1 -> Plus5/3
  Constant19/1 -> Product17/1
  Product17/1 -> Plus7/1
  Constant11/1 -> Product18/3
  Constant9/1 -> Product5/1
  Product5/1 -> Plus5/1
  [Fz] -> Product5/2
  [Fz] -> Product18/2
  Fz/1 -> Gain10/1
  Gain10/1 -> [Fz]
  Plus5/1 -> [V_lat]
  [V_lat] -> Plus4/2
  Abs/1 -> Minus1/1
  Minus1/1 -> Peak/1
  [V_lat] -> Minus1/2

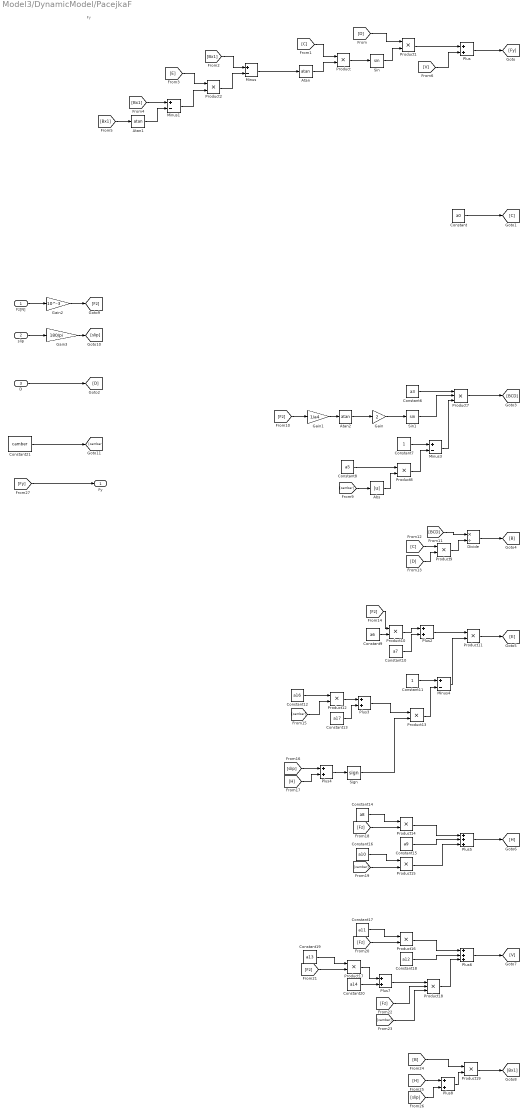
== system Model3/DynamicModel/PacejkaF ==
  note: Fy
  Fz[N] : Inport  Unit=N
  slip : Inport  Port=2  Unit=rad
  D : Inport  Port=3
  Abs : Abs
  Atan : Trigonometry  Operator=atan
  Atan1 : Trigonometry  Operator=atan
  Atan2 : Trigonometry  Operator=atan
  Constant : Constant  Value=a0
  Constant10 : Constant  Value=a7
  Constant11 : Constant
  Constant12 : Constant  Value=a16
  Constant13 : Constant  Value=a17
  Constant14 : Constant  Value=a8
  Constant15 : Constant  Value=a9
  Constant16 : Constant  Value=a10
  Constant17 : Constant  Value=a11
  Constant18 : Constant  Value=a12
  Constant19 : Constant  Value=a13
  Constant20 : Constant  Value=a14
  Constant21 : Constant  Value=camber
  Constant6 : Constant  Value=a3
  Constant7 : Constant
  Constant8 : Constant  Value=a5
  Constant9 : Constant  Value=a6
  Divide : Product  Inputs=*/
  Gain : Gain  Gain=2
  Gain1 : Gain  Gain=1/a4
  Gain2 : Gain  Gain=10^-3
  Gain3 : Gain  Gain=180/pi
  Minus{,1,3..4} (4 alike) : Sum  Inputs=+-
  Plus{,2..4,7..8} (6 alike) : Sum
  Plus5 : Sum  Inputs=+++
  Plus6 : Sum  Inputs=+++
  Product{,1..2,8..17,19} (14 alike) : Product
  Product18 : Product  Inputs=3
  Product7 : Product  Inputs=3
  Sign : Signum  ZeroCross=off
  Sin : Trigonometry
  Sin1 : Trigonometry
  Fy : Outport  Unit=N
  wires:
  Product/1 -> Sin/1
  Product2/1 -> Minus/2
  slip/1 -> Gain3/1
  Minus3/1 -> Product7/3
  Product15/1 -> Plus5/3
  Abs/1 -> Product8/2
  Constant14/1 -> Product14/1
  Gain2/1 -> [Fz]
  Constant/1 -> [C]
  Atan/1 -> Product/2
  [Fy] -> Fy/1
  Gain1/1 -> Atan2/1
  [B] -> Product19/1
  [Fz] -> Product14/2
  [Bx1] -> Minus/1
  [Fz] -> Product18/2
  Gain3/1 -> [slip]
  Gain/1 -> Sin1/1
  [Fz] -> Product10/1
  [slip] -> Plus8/2
  Plus6/1 -> [V]
  Plus2/1 -> Product11/1
  [D] -> Product1/1
  Plus5/1 -> [H]
  Minus4/1 -> Product11/2
  Minus/1 -> Atan/1
  Constant6/1 -> Product7/1
  [camber] -> Product12/2
  [V] -> Plus/2
  [C] -> Product/1
  Product19/1 -> [Bx1]
  Fz[N]/1 -> Gain2/1
  Constant21/1 -> [camber]
  Product16/1 -> Plus6/1
  Constant7/1 -> Minus3/1
  [Fz] -> Product17/2
  Product14/1 -> Plus5/1
  [BCD] -> Divide/1
  Constant20/1 -> Plus7/2
  Sin/1 -> Product1/2
  Sign/1 -> Product13/2
  Product7/1 -> [BCD]
  [camber] -> Abs/1
  Plus7/1 -> Product18/1
  Constant15/1 -> Plus5/2
  Product12/1 -> Plus3/1
  Constant18/1 -> Plus6/2
  Product11/1 -> [E]
  [Bx1] -> Minus1/1
  [Fz] -> Gain1/1
  Plus/1 -> [Fy]
  Divide/1 -> [B]
  Constant16/1 -> Product15/1
  [H] -> Plus8/1
  Atan2/1 -> Gain/1
  Plus3/1 -> Product13/1
  Constant17/1 -> Product16/1
  Product17/1 -> Plus7/1
  Product18/1 -> Plus6/3
  Constant13/1 -> Plus3/2
  Product10/1 -> Plus2/1
  Sin1/1 -> Product7/2
  [Fz] -> Product16/2
  [Bx1] -> Atan1/1
  [camber] -> Product18/3
  Minus1/1 -> Product2/2
  [C] -> Product9/1
  [camber] -> Product15/2
  Constant9/1 -> Product10/2
  [D] -> Product9/2
  Atan1/1 -> Minus1/2
  Constant19/1 -> Product17/1
  Product13/1 -> Minus4/2
  Product1/1 -> Plus/1
  D/1 -> [D]
  Plus8/1 -> Product19/2
  [E] -> Product2/1
  Constant11/1 -> Minus4/1
  Constant10/1 -> Plus2/2
  Constant12/1 -> Product12/1
  Product8/1 -> Minus3/2
  Constant8/1 -> Product8/1
  Product9/1 -> Divide/2
  [H] -> Plus4/2
  Plus4/1 -> Sign/1
  [slip] -> Plus4/1

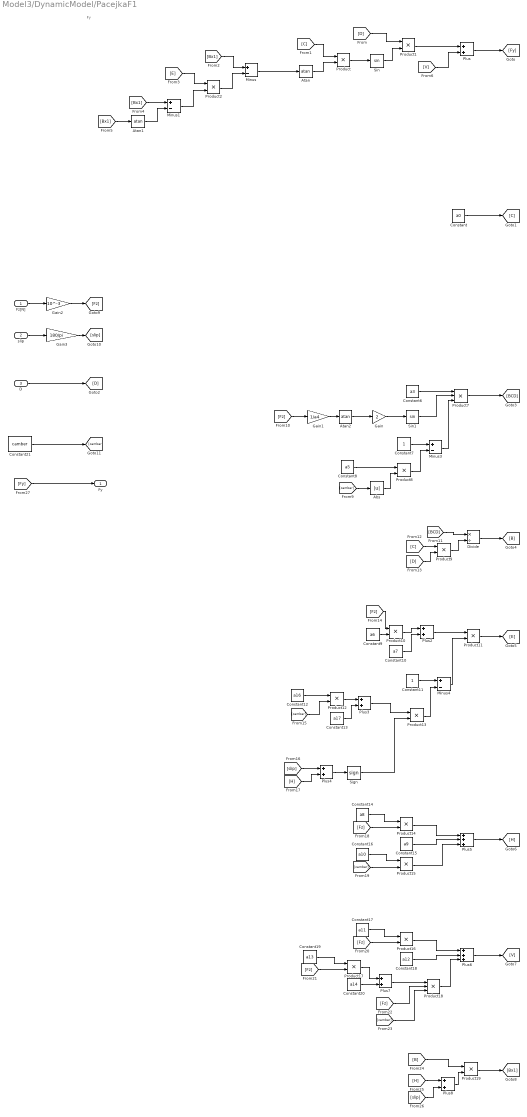
== system Model3/DynamicModel/PacejkaF1 ==
  note: Fy
  Fz[N] : Inport  Unit=N
  slip : Inport  Port=2  Unit=rad
  D : Inport  Port=3
  Abs : Abs
  Atan : Trigonometry  Operator=atan
  Atan1 : Trigonometry  Operator=atan
  Atan2 : Trigonometry  Operator=atan
  Constant : Constant  Value=a0
  Constant10 : Constant  Value=a7
  Constant11 : Constant
  Constant12 : Constant  Value=a16
  Constant13 : Constant  Value=a17
  Constant14 : Constant  Value=a8
  Constant15 : Constant  Value=a9
  Constant16 : Constant  Value=a10
  Constant17 : Constant  Value=a11
  Constant18 : Constant  Value=a12
  Constant19 : Constant  Value=a13
  Constant20 : Constant  Value=a14
  Constant21 : Constant  Value=camber
  Constant6 : Constant  Value=a3
  Constant7 : Constant
  Constant8 : Constant  Value=a5
  Constant9 : Constant  Value=a6
  Divide : Product  Inputs=*/
  Gain : Gain  Gain=2
  Gain1 : Gain  Gain=1/a4
  Gain2 : Gain  Gain=10^-3
  Gain3 : Gain  Gain=180/pi
  Minus{,1,3..4} (4 alike) : Sum  Inputs=+-
  Plus{,2..4,7..8} (6 alike) : Sum
  Plus5 : Sum  Inputs=+++
  Plus6 : Sum  Inputs=+++
  Product{,1..2,8..17,19} (14 alike) : Product
  Product18 : Product  Inputs=3
  Product7 : Product  Inputs=3
  Sign : Signum  ZeroCross=off
  Sin : Trigonometry
  Sin1 : Trigonometry
  Fy : Outport  Unit=N
  wires:
  Product/1 -> Sin/1
  Product2/1 -> Minus/2
  slip/1 -> Gain3/1
  Minus3/1 -> Product7/3
  Product15/1 -> Plus5/3
  Abs/1 -> Product8/2
  Constant14/1 -> Product14/1
  Gain2/1 -> [Fz]
  Constant/1 -> [C]
  Atan/1 -> Product/2
  [Fy] -> Fy/1
  Gain1/1 -> Atan2/1
  [B] -> Product19/1
  [Fz] -> Product14/2
  [Bx1] -> Minus/1
  [Fz] -> Product18/2
  Gain3/1 -> [slip]
  Gain/1 -> Sin1/1
  [Fz] -> Product10/1
  [slip] -> Plus8/2
  Plus6/1 -> [V]
  Plus2/1 -> Product11/1
  [D] -> Product1/1
  Plus5/1 -> [H]
  Minus4/1 -> Product11/2
  Minus/1 -> Atan/1
  Constant6/1 -> Product7/1
  [camber] -> Product12/2
  [V] -> Plus/2
  [C] -> Product/1
  Product19/1 -> [Bx1]
  Fz[N]/1 -> Gain2/1
  Constant21/1 -> [camber]
  Product16/1 -> Plus6/1
  Constant7/1 -> Minus3/1
  [Fz] -> Product17/2
  Product14/1 -> Plus5/1
  [BCD] -> Divide/1
  Constant20/1 -> Plus7/2
  Sin/1 -> Product1/2
  Sign/1 -> Product13/2
  Product7/1 -> [BCD]
  [camber] -> Abs/1
  Plus7/1 -> Product18/1
  Constant15/1 -> Plus5/2
  Product12/1 -> Plus3/1
  Constant18/1 -> Plus6/2
  Product11/1 -> [E]
  [Bx1] -> Minus1/1
  [Fz] -> Gain1/1
  Plus/1 -> [Fy]
  Divide/1 -> [B]
  Constant16/1 -> Product15/1
  [H] -> Plus8/1
  Atan2/1 -> Gain/1
  Plus3/1 -> Product13/1
  Constant17/1 -> Product16/1
  Product17/1 -> Plus7/1
  Product18/1 -> Plus6/3
  Constant13/1 -> Plus3/2
  Product10/1 -> Plus2/1
  Sin1/1 -> Product7/2
  [Fz] -> Product16/2
  [Bx1] -> Atan1/1
  [camber] -> Product18/3
  Minus1/1 -> Product2/2
  [C] -> Product9/1
  [camber] -> Product15/2
  Constant9/1 -> Product10/2
  [D] -> Product9/2
  Atan1/1 -> Minus1/2
  Constant19/1 -> Product17/1
  Product13/1 -> Minus4/2
  Product1/1 -> Plus/1
  D/1 -> [D]
  Plus8/1 -> Product19/2
  [E] -> Product2/1
  Constant11/1 -> Minus4/1
  Constant10/1 -> Plus2/2
  Constant12/1 -> Product12/1
  Product8/1 -> Minus3/2
  Constant8/1 -> Product8/1
  Product9/1 -> Divide/2
  [H] -> Plus4/2
  Plus4/1 -> Sign/1
  [slip] -> Plus4/1

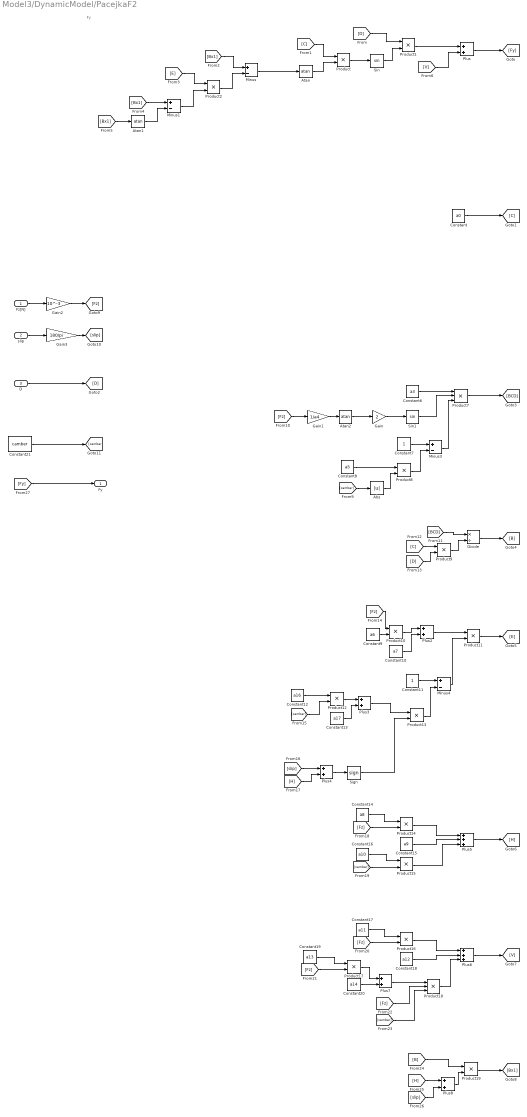
== system Model3/DynamicModel/PacejkaF2 ==
  note: Fy
  Fz[N] : Inport  Unit=N
  slip : Inport  Port=2  Unit=rad
  D : Inport  Port=3
  Abs : Abs
  Atan : Trigonometry  Operator=atan
  Atan1 : Trigonometry  Operator=atan
  Atan2 : Trigonometry  Operator=atan
  Constant : Constant  Value=a0
  Constant10 : Constant  Value=a7
  Constant11 : Constant
  Constant12 : Constant  Value=a16
  Constant13 : Constant  Value=a17
  Constant14 : Constant  Value=a8
  Constant15 : Constant  Value=a9
  Constant16 : Constant  Value=a10
  Constant17 : Constant  Value=a11
  Constant18 : Constant  Value=a12
  Constant19 : Constant  Value=a13
  Constant20 : Constant  Value=a14
  Constant21 : Constant  Value=camber
  Constant6 : Constant  Value=a3
  Constant7 : Constant
  Constant8 : Constant  Value=a5
  Constant9 : Constant  Value=a6
  Divide : Product  Inputs=*/
  Gain : Gain  Gain=2
  Gain1 : Gain  Gain=1/a4
  Gain2 : Gain  Gain=10^-3
  Gain3 : Gain  Gain=180/pi
  Minus{,1,3..4} (4 alike) : Sum  Inputs=+-
  Plus{,2..4,7..8} (6 alike) : Sum
  Plus5 : Sum  Inputs=+++
  Plus6 : Sum  Inputs=+++
  Product{,1..2,8..17,19} (14 alike) : Product
  Product18 : Product  Inputs=3
  Product7 : Product  Inputs=3
  Sign : Signum  ZeroCross=off
  Sin : Trigonometry
  Sin1 : Trigonometry
  Fy : Outport  Unit=N
  wires:
  Product/1 -> Sin/1
  Product2/1 -> Minus/2
  slip/1 -> Gain3/1
  Minus3/1 -> Product7/3
  Product15/1 -> Plus5/3
  Abs/1 -> Product8/2
  Constant14/1 -> Product14/1
  Gain2/1 -> [Fz]
  Constant/1 -> [C]
  Atan/1 -> Product/2
  [Fy] -> Fy/1
  Gain1/1 -> Atan2/1
  [B] -> Product19/1
  [Fz] -> Product14/2
  [Bx1] -> Minus/1
  [Fz] -> Product18/2
  Gain3/1 -> [slip]
  Gain/1 -> Sin1/1
  [Fz] -> Product10/1
  [slip] -> Plus8/2
  Plus6/1 -> [V]
  Plus2/1 -> Product11/1
  [D] -> Product1/1
  Plus5/1 -> [H]
  Minus4/1 -> Product11/2
  Minus/1 -> Atan/1
  Constant6/1 -> Product7/1
  [camber] -> Product12/2
  [V] -> Plus/2
  [C] -> Product/1
  Product19/1 -> [Bx1]
  Fz[N]/1 -> Gain2/1
  Constant21/1 -> [camber]
  Product16/1 -> Plus6/1
  Constant7/1 -> Minus3/1
  [Fz] -> Product17/2
  Product14/1 -> Plus5/1
  [BCD] -> Divide/1
  Constant20/1 -> Plus7/2
  Sin/1 -> Product1/2
  Sign/1 -> Product13/2
  Product7/1 -> [BCD]
  [camber] -> Abs/1
  Plus7/1 -> Product18/1
  Constant15/1 -> Plus5/2
  Product12/1 -> Plus3/1
  Constant18/1 -> Plus6/2
  Product11/1 -> [E]
  [Bx1] -> Minus1/1
  [Fz] -> Gain1/1
  Plus/1 -> [Fy]
  Divide/1 -> [B]
  Constant16/1 -> Product15/1
  [H] -> Plus8/1
  Atan2/1 -> Gain/1
  Plus3/1 -> Product13/1
  Constant17/1 -> Product16/1
  Product17/1 -> Plus7/1
  Product18/1 -> Plus6/3
  Constant13/1 -> Plus3/2
  Product10/1 -> Plus2/1
  Sin1/1 -> Product7/2
  [Fz] -> Product16/2
  [Bx1] -> Atan1/1
  [camber] -> Product18/3
  Minus1/1 -> Product2/2
  [C] -> Product9/1
  [camber] -> Product15/2
  Constant9/1 -> Product10/2
  [D] -> Product9/2
  Atan1/1 -> Minus1/2
  Constant19/1 -> Product17/1
  Product13/1 -> Minus4/2
  Product1/1 -> Plus/1
  D/1 -> [D]
  Plus8/1 -> Product19/2
  [E] -> Product2/1
  Constant11/1 -> Minus4/1
  Constant10/1 -> Plus2/2
  Constant12/1 -> Product12/1
  Product8/1 -> Minus3/2
  Constant8/1 -> Product8/1
  Product9/1 -> Divide/2
  [H] -> Plus4/2
  Plus4/1 -> Sign/1
  [slip] -> Plus4/1

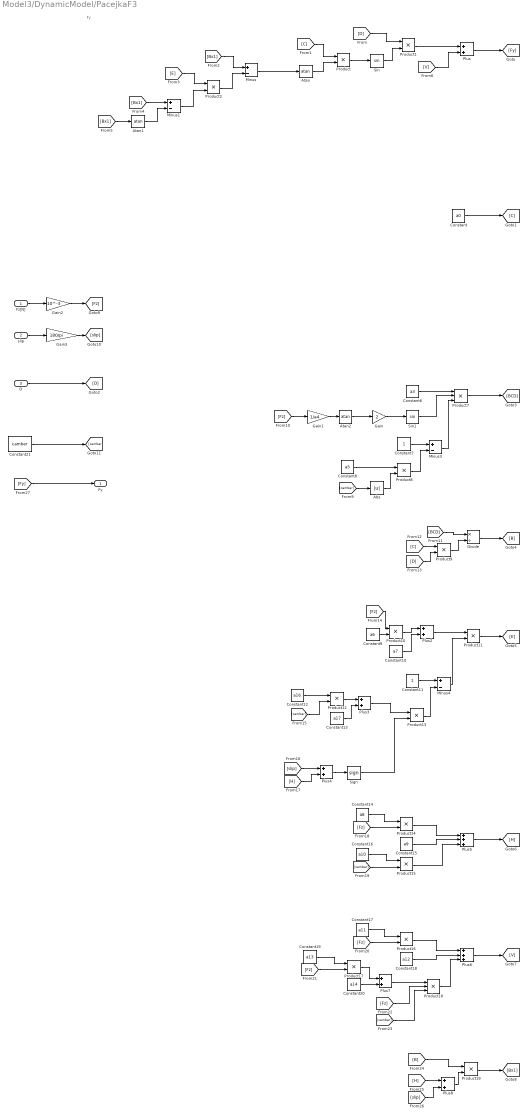
== system Model3/DynamicModel/PacejkaF3 ==
  note: Fy
  Fz[N] : Inport  Unit=N
  slip : Inport  Port=2  Unit=rad
  D : Inport  Port=3
  Abs : Abs
  Atan : Trigonometry  Operator=atan
  Atan1 : Trigonometry  Operator=atan
  Atan2 : Trigonometry  Operator=atan
  Constant : Constant  Value=a0
  Constant10 : Constant  Value=a7
  Constant11 : Constant
  Constant12 : Constant  Value=a16
  Constant13 : Constant  Value=a17
  Constant14 : Constant  Value=a8
  Constant15 : Constant  Value=a9
  Constant16 : Constant  Value=a10
  Constant17 : Constant  Value=a11
  Constant18 : Constant  Value=a12
  Constant19 : Constant  Value=a13
  Constant20 : Constant  Value=a14
  Constant21 : Constant  Value=camber
  Constant6 : Constant  Value=a3
  Constant7 : Constant
  Constant8 : Constant  Value=a5
  Constant9 : Constant  Value=a6
  Divide : Product  Inputs=*/
  Gain : Gain  Gain=2
  Gain1 : Gain  Gain=1/a4
  Gain2 : Gain  Gain=10^-3
  Gain3 : Gain  Gain=180/pi
  Minus{,1,3..4} (4 alike) : Sum  Inputs=+-
  Plus{,2..4,7..8} (6 alike) : Sum
  Plus5 : Sum  Inputs=+++
  Plus6 : Sum  Inputs=+++
  Product{,1..2,8..17,19} (14 alike) : Product
  Product18 : Product  Inputs=3
  Product7 : Product  Inputs=3
  Sign : Signum  ZeroCross=off
  Sin : Trigonometry
  Sin1 : Trigonometry
  Fy : Outport  Unit=N
  wires:
  Product/1 -> Sin/1
  Product2/1 -> Minus/2
  slip/1 -> Gain3/1
  Minus3/1 -> Product7/3
  Product15/1 -> Plus5/3
  Abs/1 -> Product8/2
  Constant14/1 -> Product14/1
  Gain2/1 -> [Fz]
  Constant/1 -> [C]
  Atan/1 -> Product/2
  [Fy] -> Fy/1
  Gain1/1 -> Atan2/1
  [B] -> Product19/1
  [Fz] -> Product14/2
  [Bx1] -> Minus/1
  [Fz] -> Product18/2
  Gain3/1 -> [slip]
  Gain/1 -> Sin1/1
  [Fz] -> Product10/1
  [slip] -> Plus8/2
  Plus6/1 -> [V]
  Plus2/1 -> Product11/1
  [D] -> Product1/1
  Plus5/1 -> [H]
  Minus4/1 -> Product11/2
  Minus/1 -> Atan/1
  Constant6/1 -> Product7/1
  [camber] -> Product12/2
  [V] -> Plus/2
  [C] -> Product/1
  Product19/1 -> [Bx1]
  Fz[N]/1 -> Gain2/1
  Constant21/1 -> [camber]
  Product16/1 -> Plus6/1
  Constant7/1 -> Minus3/1
  [Fz] -> Product17/2
  Product14/1 -> Plus5/1
  [BCD] -> Divide/1
  Constant20/1 -> Plus7/2
  Sin/1 -> Product1/2
  Sign/1 -> Product13/2
  Product7/1 -> [BCD]
  [camber] -> Abs/1
  Plus7/1 -> Product18/1
  Constant15/1 -> Plus5/2
  Product12/1 -> Plus3/1
  Constant18/1 -> Plus6/2
  Product11/1 -> [E]
  [Bx1] -> Minus1/1
  [Fz] -> Gain1/1
  Plus/1 -> [Fy]
  Divide/1 -> [B]
  Constant16/1 -> Product15/1
  [H] -> Plus8/1
  Atan2/1 -> Gain/1
  Plus3/1 -> Product13/1
  Constant17/1 -> Product16/1
  Product17/1 -> Plus7/1
  Product18/1 -> Plus6/3
  Constant13/1 -> Plus3/2
  Product10/1 -> Plus2/1
  Sin1/1 -> Product7/2
  [Fz] -> Product16/2
  [Bx1] -> Atan1/1
  [camber] -> Product18/3
  Minus1/1 -> Product2/2
  [C] -> Product9/1
  [camber] -> Product15/2
  Constant9/1 -> Product10/2
  [D] -> Product9/2
  Atan1/1 -> Minus1/2
  Constant19/1 -> Product17/1
  Product13/1 -> Minus4/2
  Product1/1 -> Plus/1
  D/1 -> [D]
  Plus8/1 -> Product19/2
  [E] -> Product2/1
  Constant11/1 -> Minus4/1
  Constant10/1 -> Plus2/2
  Constant12/1 -> Product12/1
  Product8/1 -> Minus3/2
  Constant8/1 -> Product8/1
  Product9/1 -> Divide/2
  [H] -> Plus4/2
  Plus4/1 -> Sign/1
  [slip] -> Plus4/1

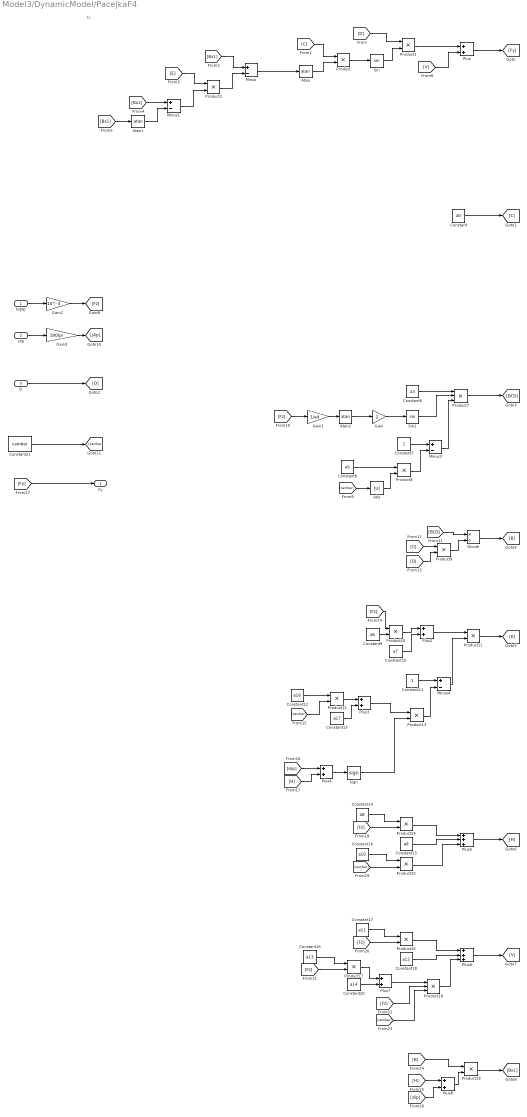
== system Model3/DynamicModel/PacejkaF4 ==
  note: Fy
  Fz[N] : Inport  Unit=N
  slip : Inport  Port=2  Unit=rad
  D : Inport  Port=3
  Abs : Abs
  Atan : Trigonometry  Operator=atan
  Atan1 : Trigonometry  Operator=atan
  Atan2 : Trigonometry  Operator=atan
  Constant : Constant  Value=a0
  Constant10 : Constant  Value=a7
  Constant11 : Constant
  Constant12 : Constant  Value=a16
  Constant13 : Constant  Value=a17
  Constant14 : Constant  Value=a8
  Constant15 : Constant  Value=a9
  Constant16 : Constant  Value=a10
  Constant17 : Constant  Value=a11
  Constant18 : Constant  Value=a12
  Constant19 : Constant  Value=a13
  Constant20 : Constant  Value=a14
  Constant21 : Constant  Value=camber
  Constant6 : Constant  Value=a3
  Constant7 : Constant
  Constant8 : Constant  Value=a5
  Constant9 : Constant  Value=a6
  Divide : Product  Inputs=*/
  Gain : Gain  Gain=2
  Gain1 : Gain  Gain=1/a4
  Gain2 : Gain  Gain=10^-3
  Gain3 : Gain  Gain=180/pi
  Minus{,1,3..4} (4 alike) : Sum  Inputs=+-
  Plus{,2..4,7..8} (6 alike) : Sum
  Plus5 : Sum  Inputs=+++
  Plus6 : Sum  Inputs=+++
  Product{,1..2,8..17,19} (14 alike) : Product
  Product18 : Product  Inputs=3
  Product7 : Product  Inputs=3
  Sign : Signum  ZeroCross=off
  Sin : Trigonometry
  Sin1 : Trigonometry
  Fy : Outport  Unit=N
  wires:
  Product/1 -> Sin/1
  Product2/1 -> Minus/2
  slip/1 -> Gain3/1
  Minus3/1 -> Product7/3
  Product15/1 -> Plus5/3
  Abs/1 -> Product8/2
  Constant14/1 -> Product14/1
  Gain2/1 -> [Fz]
  Constant/1 -> [C]
  Atan/1 -> Product/2
  [Fy] -> Fy/1
  Gain1/1 -> Atan2/1
  [B] -> Product19/1
  [Fz] -> Product14/2
  [Bx1] -> Minus/1
  [Fz] -> Product18/2
  Gain3/1 -> [slip]
  Gain/1 -> Sin1/1
  [Fz] -> Product10/1
  [slip] -> Plus8/2
  Plus6/1 -> [V]
  Plus2/1 -> Product11/1
  [D] -> Product1/1
  Plus5/1 -> [H]
  Minus4/1 -> Product11/2
  Minus/1 -> Atan/1
  Constant6/1 -> Product7/1
  [camber] -> Product12/2
  [V] -> Plus/2
  [C] -> Product/1
  Product19/1 -> [Bx1]
  Fz[N]/1 -> Gain2/1
  Constant21/1 -> [camber]
  Product16/1 -> Plus6/1
  Constant7/1 -> Minus3/1
  [Fz] -> Product17/2
  Product14/1 -> Plus5/1
  [BCD] -> Divide/1
  Constant20/1 -> Plus7/2
  Sin/1 -> Product1/2
  Sign/1 -> Product13/2
  Product7/1 -> [BCD]
  [camber] -> Abs/1
  Plus7/1 -> Product18/1
  Constant15/1 -> Plus5/2
  Product12/1 -> Plus3/1
  Constant18/1 -> Plus6/2
  Product11/1 -> [E]
  [Bx1] -> Minus1/1
  [Fz] -> Gain1/1
  Plus/1 -> [Fy]
  Divide/1 -> [B]
  Constant16/1 -> Product15/1
  [H] -> Plus8/1
  Atan2/1 -> Gain/1
  Plus3/1 -> Product13/1
  Constant17/1 -> Product16/1
  Product17/1 -> Plus7/1
  Product18/1 -> Plus6/3
  Constant13/1 -> Plus3/2
  Product10/1 -> Plus2/1
  Sin1/1 -> Product7/2
  [Fz] -> Product16/2
  [Bx1] -> Atan1/1
  [camber] -> Product18/3
  Minus1/1 -> Product2/2
  [C] -> Product9/1
  [camber] -> Product15/2
  Constant9/1 -> Product10/2
  [D] -> Product9/2
  Atan1/1 -> Minus1/2
  Constant19/1 -> Product17/1
  Product13/1 -> Minus4/2
  Product1/1 -> Plus/1
  D/1 -> [D]
  Plus8/1 -> Product19/2
  [E] -> Product2/1
  Constant11/1 -> Minus4/1
  Constant10/1 -> Plus2/2
  Constant12/1 -> Product12/1
  Product8/1 -> Minus3/2
  Constant8/1 -> Product8/1
  Product9/1 -> Divide/2
  [H] -> Plus4/2
  Plus4/1 -> Sign/1
  [slip] -> Plus4/1

== matlab function Model3/Subsystem/MATLAB Function1 ==
  data: clock input; steer output
function steer = steerCalculation(clock)

if clock <= 14
    steer = 0;
elseif clock > 14 && clock <= 15
    steer = 0.005;
elseif clock > 15 && clock <= 20
    steer = 0.025;
elseif clock > 20 && clock <= 22
    steer = 0.02;
elseif clock > 22 && clock <= 25
    steer = 0;
elseif clock > 25 && clock <= 26
    steer = 0.03;
elseif clock > 26 && clock <= 33
    steer = 0.01;
elseif clock > 33 && clock <= 35
    steer = -0.02;
elseif clock > 35 && clock <= 40
    steer = 0;
elseif clock > 40 && clock <= 41
    steer = 0.03;
elseif clock > 41 && clock <= 43
    steer = 0.02;
elseif clock > 43 && clock <= 50
    steer = 0.01;
elseif clock > 50 && clock <= 53
    steer = 0.02;
elseif clock > 53 && clock <= 55
    steer = 0.01;
elseif clock > 55 && clock <= 57
    steer = 0.006;
elseif clock > 57 && clock <= 60
    steer = 0;
else
    steer = 0;
end

== matlab function Model3/Subsystem/MATLAB Function ==
  data: clock input; force output
function force = forceCalculatation(clock)

if clock <= 10
    force = 2000;
elseif clock > 10 && clock <= 20
    force = 400;
elseif clock > 20 && clock <= 30
    force = -500;
elseif clock > 30 && clock <= 40
    force = 500;
elseif clock > 40 && clock <= 42
    force = 1500;
elseif clock > 42 && clock <= 44
    force = -750;
elseif clock > 44 && clock <= 46
    force = 500;
elseif clock > 57 && clock <= 90
    force = 1500;
else
    force = 500;
end

== matlab function Model3/DynamicModel/FindBankingData ==
  data: x input; res output; y input; curveCenters input; bankingAngle input
function res = findBannkingData (x, y, curveCenters, bankingAngle)

if  ...
    (x > curveCenters(1,1) && y < curveCenters(1,2)) || ... %check if in the first curve
    (x > curveCenters(2,1) && y > curveCenters(2,2)) || ... %check if in the second curve
    (x < curveCenters(3,1) && y > curveCenters(3,2)) || ... %check if in the third curve
    (x < curveCenters(4,1) && y < curveCenters(4,2))        %check if in the fourth curve
        
    res = bankingAngle;
    %res = 0;
 
%default result for straights
else 
    res = 0;
end
